simulink model "Md31StEnCtrl"  (R2018b)
settings: Solver=FixedStepDiscrete  StartTime=0.0  StopTime=10.0  FixedStep=0.01  RelTol=1e-3  EnableMultiTasking=on
undefined symbols (not defined in the file or in its folder): data, KeSMSuFirstRwStFwdBkwdPosDelta_Val, KeSMSw4SSecRwRtStLgrstOtwdInwdClosePos1_Val, KeSMSw4SSecRwRtStLgrstUpwdDnwdClosePos1_Val, KeSMSw4SSecRwRtStLgrstUpwdDnwdClosePos2_Val, PassStBkReclnEn_Clear, PassStBkReclnEn_Set, PassStCshnFldEn_Clear, PassStCshnFldEn_Set, PassStFwdBkwdEn_Clear, PassStFwdBkwdEn_Set, SecRwRtStLgrstInwdOtwdEn_Clear, SecRwRtStLgrstInwdOtwdEn_Set, SecRwRtStLgrstUpwdDnwdEn_Clear, SecRwRtStLgrstUpwdDnwdEn_Set
libraries: simulink x2
settings Model: Creator=sn55gm  LastModifiedBy=sn55gm
settings Model: ModifiedHistory=|
  | 2025.7.15 二排腿托enset修复
  | 2025.09.03 前后或折叠都fail结束执行
settings DataIOCC: SaveFormat=StructureWithTime
settings OptimizationCC: DefaultParameterBehavior=Inlined  UseDivisionForNetSlopeComputation=on  UseFloatMulNetSlope=on  InlineInvariantSignals=on  PassReuseOutputArgsAs=Individual arguments  ZeroExternalMemoryAtStartup=off  ZeroInternalMemoryAtStartup=off  NoFixptDivByZeroProtection=on  EfficientFloat2IntCast=on  LifeSpan=1  OptimizeBlockOrder=speed  DifferentSizesBufferReuse=on
settings DebuggingCC: ParameterTunabilityLossMsg=error
settings HardwareCC: ProdLongLongMode=on
settings SFSimCC: MATLABDynamicMemAlloc=off
settings RTWCC: SystemTargetFile=autosar.tlc  GenCodeOnly=on  TemplateMakefile=ert_default_tmf  Description=AUTOSAR  GenerateReport=on  IncludeHyperlinkInReport=on  LaunchReport=on  GenerateTraceInfo=on  GenerateTraceReport=on  GenerateTraceReportSl=on  GenerateTraceReportSf=on  GenerateTraceReportEml=on  GenerateCodeMetricsReport=on
settings CodeAppCC: ForceParamTrailComments=on  IgnoreCustomStorageClasses=off  OperatorAnnotations=on  SimulinkDataObjDesc=on  SFDataObjDesc=on  CustomSymbolStrGlobalVar=rt$N$M  CustomSymbolStrType=$N$M  CustomSymbolStrFcn=$N$M$F  CustomSymbolStrMacro=$N$M  InsertBlockDesc=on
settings STFCustomTargetCC: TargetLangStandard=C99 (ISO)  MultiwordLength=256  ParMdlRefBuildCompliant=on  CompOptLevelCompliant=on  IncludeMdlTerminateFcn=off  CombineOutputUpdateFcns=on  CombineSignalStateStructs=on  SuppressErrorStatus=on  ERTCustomFileBanners=on  SupportAbsoluteTime=off  SupportNonFinite=off  SupportComplex=off  SupportContinuousTime=off  SupportNonInlinedSFcns=off  RemoveResetFunc=on  MATLABClassNameForMDSCustomization=Simulink.SoftwareTarget.ERTCustomization  AutosarCompliant=on  UseToolchainInfoCompliant=on  LookupTableObjectStructAxisOrder=2,1,3,4,...  LUTObjectStructOrderEvenSpacing=Size,Table,Breakpoints  SystemTargetFile=autosar.tlc
settings ERTTargetCC: TargetLangStandard=C99 (ISO)  ConcurrentExecutionCompliant=off  IncludeMdlTerminateFcn=off  CombineSignalStateStructs=on  SuppressErrorStatus=on  SupportAbsoluteTime=off  SupportNonFinite=off  SupportComplex=off  ModelStepFunctionPrototypeControlCompliant=off  CPPClassGenCompliant=off  AutosarCompliant=on  LookupTableObjectStructAxisOrder=2,1,3,4,...  LUTObjectStructOrderEvenSpacing=Size,Table,Breakpoints  InlinedParameterPlacement=NonHierarchical  ERTCustomFileTemplate=example_file_process.tlc  ERTFilePackagingFormat=CompactWithDataFile

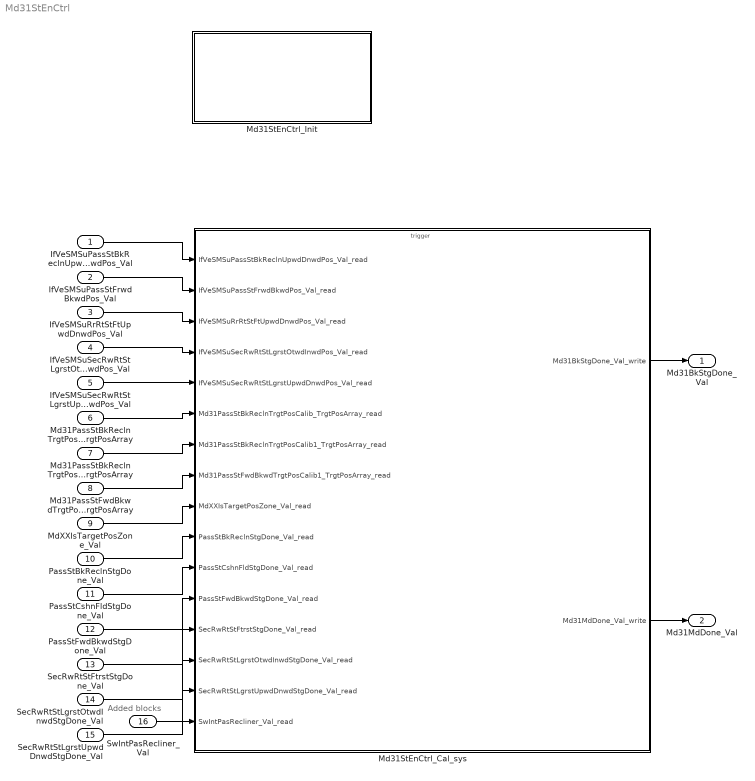
== system Md31StEnCtrl ==
  note: Added blocks
  IfVeSMSuPassStBkReclnUpwdDnwdPos_Val : Inport  OutDataTypeStr=uint16  PortDimensions=1
  IfVeSMSuPassStFrwdBkwdPos_Val : Inport  Port=2  OutDataTypeStr=uint16  PortDimensions=1
  IfVeSMSuRrRtStFtUpwdDnwdPos_Val : Inport  Port=3  OutDataTypeStr=uint16  PortDimensions=1
  IfVeSMSuSecRwRtStLgrstOtwdInwdPos_Val : Inport  Port=4  OutDataTypeStr=uint16  PortDimensions=1
  IfVeSMSuSecRwRtStLgrstUpwdDnwdPos_Val : Inport  Port=5  OutDataTypeStr=uint16  PortDimensions=1
  Md31PassStBkReclnTrgtPosCalib_TrgtPosArray : Inport  Description=|  Port=6  OutDataTypeStr=uint16  PortDimensions=3
      | 0:Pos
      | 1:Max
      | 2:Min
  Md31PassStBkReclnTrgtPosCalib1_TrgtPosArray : Inport  Description=|  Port=7  OutDataTypeStr=uint16  PortDimensions=3
      | 0:Pos
      | 1:Max
      | 2:Min
  Md31PassStFwdBkwdTrgtPosCalib1_TrgtPosArray : Inport  Description=|  Port=8  OutDataTypeStr=uint16  PortDimensions=3
      | 0:Pos
      | 1:Max
      | 2:Min
  MdXXIsTargetPosZone_Val : Inport  Port=9  OutDataTypeStr=uint32  PortDimensions=1
  PassStBkReclnStgDone_Val : Inport  Port=10  OutDataTypeStr=boolean  PortDimensions=1
  PassStCshnFldStgDone_Val : Inport  Port=11  OutDataTypeStr=boolean  PortDimensions=1
  PassStFwdBkwdStgDone_Val : Inport  Port=12  OutDataTypeStr=boolean  PortDimensions=1
  SecRwRtStFtrstStgDone_Val : Inport  Port=13  OutDataTypeStr=boolean  PortDimensions=1
  SecRwRtStLgrstOtwdInwdStgDone_Val : Inport  Port=14  OutDataTypeStr=boolean  PortDimensions=1
  SecRwRtStLgrstUpwdDnwdStgDone_Val : Inport  Port=15  OutDataTypeStr=boolean  PortDimensions=1
  SwIntPasRecliner_Val : Inport  Port=16  OutDataTypeStr=boolean  PortDimensions=1
  Md31StEnCtrl_Cal_sys : Subsystem
  Md31StEnCtrl_Init : Subsystem
  Md31BkStgDone_Val : Outport  OutDataTypeStr=boolean  PortDimensions=1
  Md31MdDone_Val : Outport  Port=2  OutDataTypeStr=uint8  PortDimensions=1
  wires:
  IfVeSMSuPassStBkReclnUpwdDnwdPos_Val/1 -> Md31StEnCtrl_Cal_sys/1(IfVeSMSuPassStBkReclnUpwdDnwdPos_Val_read)
  IfVeSMSuPassStFrwdBkwdPos_Val/1 -> Md31StEnCtrl_Cal_sys/2(IfVeSMSuPassStFrwdBkwdPos_Val_read)
  IfVeSMSuRrRtStFtUpwdDnwdPos_Val/1 -> Md31StEnCtrl_Cal_sys/3(IfVeSMSuRrRtStFtUpwdDnwdPos_Val_read)
  IfVeSMSuSecRwRtStLgrstOtwdInwdPos_Val/1 -> Md31StEnCtrl_Cal_sys/4(IfVeSMSuSecRwRtStLgrstOtwdInwdPos_Val_read)
  IfVeSMSuSecRwRtStLgrstUpwdDnwdPos_Val/1 -> Md31StEnCtrl_Cal_sys/5(IfVeSMSuSecRwRtStLgrstUpwdDnwdPos_Val_read)
  Md31PassStBkReclnTrgtPosCalib_TrgtPosArray/1 -> Md31StEnCtrl_Cal_sys/6(Md31PassStBkReclnTrgtPosCalib_TrgtPosArray_read)
  Md31PassStBkReclnTrgtPosCalib1_TrgtPosArray/1 -> Md31StEnCtrl_Cal_sys/7(Md31PassStBkReclnTrgtPosCalib1_TrgtPosArray_read)
  Md31PassStFwdBkwdTrgtPosCalib1_TrgtPosArray/1 -> Md31StEnCtrl_Cal_sys/8(Md31PassStFwdBkwdTrgtPosCalib1_TrgtPosArray_read)
  MdXXIsTargetPosZone_Val/1 -> Md31StEnCtrl_Cal_sys/9(MdXXIsTargetPosZone_Val_read)
  PassStBkReclnStgDone_Val/1 -> Md31StEnCtrl_Cal_sys/10(PassStBkReclnStgDone_Val_read)
  PassStCshnFldStgDone_Val/1 -> Md31StEnCtrl_Cal_sys/11(PassStCshnFldStgDone_Val_read)
  PassStFwdBkwdStgDone_Val/1 -> Md31StEnCtrl_Cal_sys/12(PassStFwdBkwdStgDone_Val_read)
  SecRwRtStFtrstStgDone_Val/1 -> Md31StEnCtrl_Cal_sys/13(SecRwRtStFtrstStgDone_Val_read)
  SecRwRtStLgrstOtwdInwdStgDone_Val/1 -> Md31StEnCtrl_Cal_sys/14(SecRwRtStLgrstOtwdInwdStgDone_Val_read)
  SecRwRtStLgrstUpwdDnwdStgDone_Val/1 -> Md31StEnCtrl_Cal_sys/15(SecRwRtStLgrstUpwdDnwdStgDone_Val_read)
  Md31StEnCtrl_Cal_sys/1(Md31BkStgDone_Val_write) -> Md31BkStgDone_Val/1
  Md31StEnCtrl_Cal_sys/2(Md31MdDone_Val_write) -> Md31MdDone_Val/1
  SwIntPasRecliner_Val/1 -> Md31StEnCtrl_Cal_sys/16(SwIntPasRecliner_Val_read)

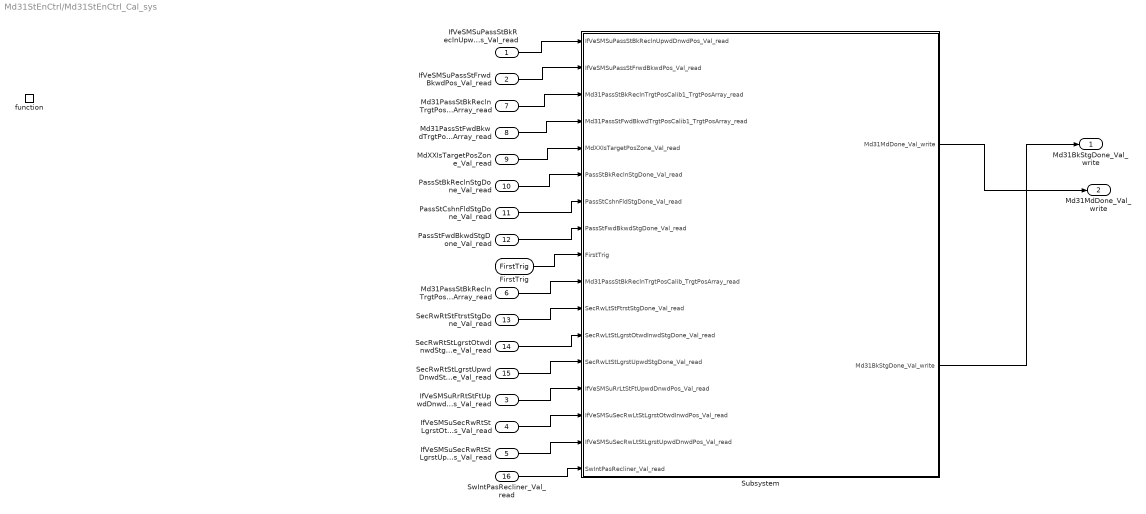
== system Md31StEnCtrl/Md31StEnCtrl_Cal_sys ==
  IfVeSMSuPassStBkReclnUpwdDnwdPos_Val_read : Inport
  IfVeSMSuPassStFrwdBkwdPos_Val_read : Inport  Port=2
  IfVeSMSuRrRtStFtUpwdDnwdPos_Val_read : Inport  Port=3
  IfVeSMSuSecRwRtStLgrstOtwdInwdPos_Val_read : Inport  Port=4
  IfVeSMSuSecRwRtStLgrstUpwdDnwdPos_Val_read : Inport  Port=5
  Md31PassStBkReclnTrgtPosCalib_TrgtPosArray_read : Inport  Port=6
  Md31PassStBkReclnTrgtPosCalib1_TrgtPosArray_read : Inport  Port=7
  Md31PassStFwdBkwdTrgtPosCalib1_TrgtPosArray_read : Inport  Port=8
  MdXXIsTargetPosZone_Val_read : Inport  Port=9
  PassStBkReclnStgDone_Val_read : Inport  Port=10
  PassStCshnFldStgDone_Val_read : Inport  Port=11
  PassStFwdBkwdStgDone_Val_read : Inport  Port=12
  SecRwRtStFtrstStgDone_Val_read : Inport  Port=13
  SecRwRtStLgrstOtwdInwdStgDone_Val_read : Inport  Port=14
  SecRwRtStLgrstUpwdDnwdStgDone_Val_read : Inport  Port=15
  SwIntPasRecliner_Val_read : Inport  Port=16
  function : TriggerPort  TriggerType=function-call  IsSimulinkFunction=on  FunctionName=Md31StEnCtrl_Cal  VariantControl=(inherit)
  Subsystem : Subsystem
  FirstTrig : ArgIn  OutDataTypeStr=boolean  ArgumentName=FirstTrig
  Md31BkStgDone_Val_write : Outport
      settings: EnsureOutportIsVirtual=on
  Md31MdDone_Val_write : Outport  Port=2
      settings: EnsureOutportIsVirtual=on
  wires:
  IfVeSMSuPassStBkReclnUpwdDnwdPos_Val_read/1 -> Subsystem/1(IfVeSMSuPassStBkReclnUpwdDnwdPos_Val_read)
  Md31PassStFwdBkwdTrgtPosCalib1_TrgtPosArray_read/1 -> Subsystem/4(Md31PassStFwdBkwdTrgtPosCalib1_TrgtPosArray_read)
  PassStBkReclnStgDone_Val_read/1 -> Subsystem/6(PassStBkReclnStgDone_Val_read)
  PassStFwdBkwdStgDone_Val_read/1 -> Subsystem/8(PassStFwdBkwdStgDone_Val_read)
  FirstTrig/1 -> Subsystem/9(FirstTrig)
  Subsystem/2(Md31BkStgDone_Val_write) -> Md31BkStgDone_Val_write/1
  Subsystem/1(Md31MdDone_Val_write) -> Md31MdDone_Val_write/1
  IfVeSMSuPassStFrwdBkwdPos_Val_read/1 -> Subsystem/2(IfVeSMSuPassStFrwdBkwdPos_Val_read)
  MdXXIsTargetPosZone_Val_read/1 -> Subsystem/5(MdXXIsTargetPosZone_Val_read)
  PassStCshnFldStgDone_Val_read/1 -> Subsystem/7(PassStCshnFldStgDone_Val_read)
  SecRwRtStFtrstStgDone_Val_read/1 -> Subsystem/11(SecRwLtStFtrstStgDone_Val_read)
  SecRwRtStLgrstOtwdInwdStgDone_Val_read/1 -> Subsystem/12(SecRwLtStLgrstOtwdInwdStgDone_Val_read)
  SecRwRtStLgrstUpwdDnwdStgDone_Val_read/1 -> Subsystem/13(SecRwLtStLgrstUpwdStgDone_Val_read)
  IfVeSMSuRrRtStFtUpwdDnwdPos_Val_read/1 -> Subsystem/14(IfVeSMSuRrLtStFtUpwdDnwdPos_Val_read)
  Md31PassStBkReclnTrgtPosCalib_TrgtPosArray_read/1 -> Subsystem/10(Md31PassStBkReclnTrgtPosCalib_TrgtPosArray_read)
  Md31PassStBkReclnTrgtPosCalib1_TrgtPosArray_read/1 -> Subsystem/3(Md31PassStBkReclnTrgtPosCalib1_TrgtPosArray_read)
  IfVeSMSuSecRwRtStLgrstOtwdInwdPos_Val_read/1 -> Subsystem/15(IfVeSMSuSecRwLtStLgrstOtwdInwdPos_Val_read)
  IfVeSMSuSecRwRtStLgrstUpwdDnwdPos_Val_read/1 -> Subsystem/16(IfVeSMSuSecRwLtStLgrstUpwdDnwdPos_Val_read)
  SwIntPasRecliner_Val_read/1 -> Subsystem/17(SwIntPasRecliner_Val_read)

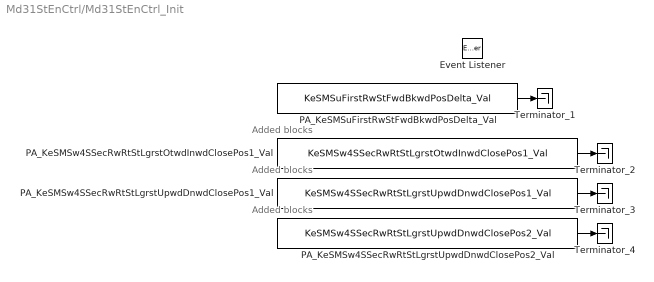
== system Md31StEnCtrl/Md31StEnCtrl_Init ==
  note: Added blocks
  note: Added blocks
  note: Added blocks
  Event Listener : EventListener  EventName=reset
  PA_KeSMSuFirstRwStFwdBkwdPosDelta_Val : Constant  Value=KeSMSuFirstRwStFwdBkwdPosDelta_Val
  PA_KeSMSw4SSecRwRtStLgrstOtwdInwdClosePos1_Val : Constant  Value=KeSMSw4SSecRwRtStLgrstOtwdInwdClosePos1_Val
  PA_KeSMSw4SSecRwRtStLgrstUpwdDnwdClosePos1_Val : Constant  Value=KeSMSw4SSecRwRtStLgrstUpwdDnwdClosePos1_Val
  PA_KeSMSw4SSecRwRtStLgrstUpwdDnwdClosePos2_Val : Constant  Value=KeSMSw4SSecRwRtStLgrstUpwdDnwdClosePos2_Val
  Terminator_{1..4} (4 alike) : Terminator
  wires:
  PA_KeSMSuFirstRwStFwdBkwdPosDelta_Val/1 -> Terminator_1/1
  PA_KeSMSw4SSecRwRtStLgrstOtwdInwdClosePos1_Val/1 -> Terminator_2/1
  PA_KeSMSw4SSecRwRtStLgrstUpwdDnwdClosePos1_Val/1 -> Terminator_3/1
  PA_KeSMSw4SSecRwRtStLgrstUpwdDnwdClosePos2_Val/1 -> Terminator_4/1

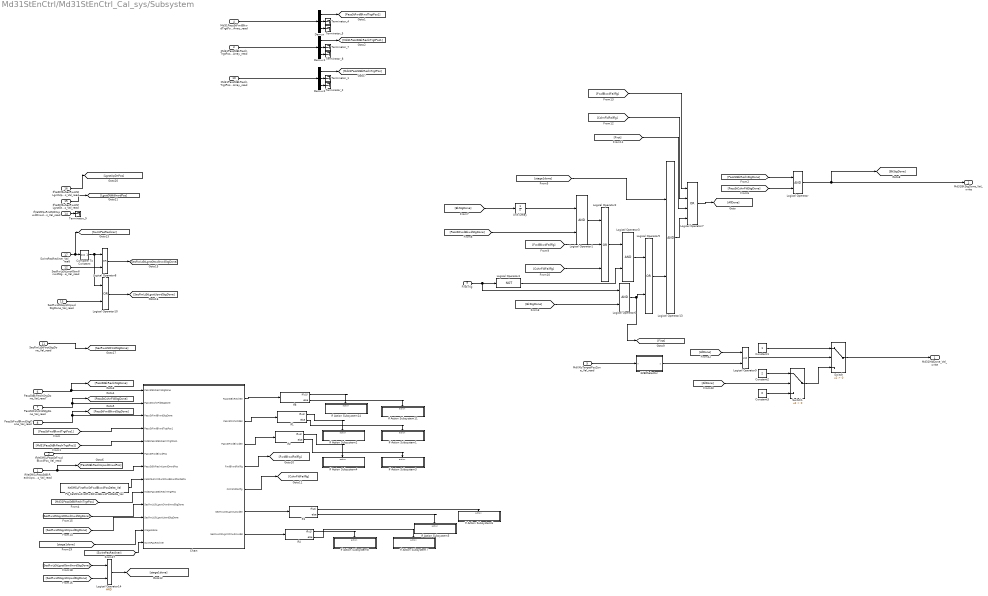
== system Md31StEnCtrl/Md31StEnCtrl_Cal_sys/Subsystem ==
  IfVeSMSuPassStBkReclnUpwdDnwdPos_Val_read : Inport
  IfVeSMSuPassStFrwdBkwdPos_Val_read : Inport  Port=2
  Md31PassStBkReclnTrgtPosCalib1_TrgtPosArray_read : Inport  Port=3
  Md31PassStFwdBkwdTrgtPosCalib1_TrgtPosArray_read : Inport  Port=4
  MdXXIsTargetPosZone_Val_read : Inport  Port=5
  PassStBkReclnStgDone_Val_read : Inport  Port=6
  PassStCshnFldStgDone_Val_read : Inport  Port=7
  PassStFwdBkwdStgDone_Val_read : Inport  Port=8
  FirstTrig : Inport  Port=9
  Md31PassStBkReclnTrgtPosCalib_TrgtPosArray_read : Inport  Port=10
  SecRwLtStFtrstStgDone_Val_read : Inport  Port=11
  SecRwLtStLgrstOtwdInwdStgDone_Val_read : Inport  Port=12
  SecRwLtStLgrstUpwdStgDone_Val_read : Inport  Port=13
  IfVeSMSuRrLtStFtUpwdDnwdPos_Val_read : Inport  Port=14
  IfVeSMSuSecRwLtStLgrstOtwdInwdPos_Val_read : Inport  Port=15
  IfVeSMSuSecRwLtStLgrstUpwdDnwdPos_Val_read : Inport  Port=16
  SwIntPasRecliner_Val_read : Inport  Port=17
  32BitSelector : Subsystem  mask(32 Bit Selector){BitNum=30}
      mask prompts: BitNum "Select Bit Number"
      mask help: Allows selection of a particular bit (0-31) out of a packed word up to 32 bits long. Output will be true if the bit number selected via the mask parameter is equal to one.
      mask TypeOptions BitNum: 0 | 1 | 2 | 3 | 4 | 5 | 6 | 7 | 8 | 9 | 10 | 11 | 12 | 13 | 14 | 15 | 16 | 17 | 18 | 19 | 20 | 21 | 22 | 23 | 24 | 25 | 26 | 27 | 28 | 29 | 30 | 31
      mask Display:
      | text(0.5, 0.8,'BIT','horizontalAlignment','center')
      | text(0.5, 0.5,'SELECTOR','horizontalAlignment','center')
      | text(0.5, 0.2,['-- Bit ',char(get_param(gcb,'BitNum')),' --'],'horizontalAlignment','center')
  Chart : Stateflow chart  TreatAsAtomicUnit=on
  Compare To Constant : simulink/Logic and Bit Operations/Compare To Constant  relop===  const=1  OutDataTypeStr=boolean
  Constant1 : Constant  OutDataTypeStr=uint8
  Constant2 : Constant  Value=2  OutDataTypeStr=uint8
  Constant3 : Constant  Value=0  OutDataTypeStr=uint8
  Demux : Demux  Outputs=3
  Demux1 : Demux  Outputs=3
  Demux2 : Demux  Outputs=3
  If Action Subsystem1 : Subsystem  TreatAsAtomicUnit=on
  If Action Subsystem11 : Subsystem  TreatAsAtomicUnit=on
  If Action Subsystem14 : Subsystem  TreatAsAtomicUnit=on
  If Action Subsystem2 : Subsystem  TreatAsAtomicUnit=on
  If Action Subsystem3 : Subsystem  TreatAsAtomicUnit=on
  If Action Subsystem4 : Subsystem  TreatAsAtomicUnit=on
  If Action Subsystem5 : Subsystem  TreatAsAtomicUnit=on
  If Action Subsystem6 : Subsystem  TreatAsAtomicUnit=on
  If Action Subsystem7 : Subsystem  TreatAsAtomicUnit=on
  If Action Subsystem8 : Subsystem  TreatAsAtomicUnit=on
  If{1..4,8} (5 alike) : If  IfExpression=u1
  Logical Operator{,1,3,6,9,13..14} (7 alike) : Logic  AllPortsSameDT=off  OutDataTypeStr=boolean
  Logical Operator10 : Logic  Operator=OR  AllPortsSameDT=off  OutDataTypeStr=boolean
  Logical Operator2 : Logic  Operator=OR  Inputs=3  AllPortsSameDT=off  OutDataTypeStr=boolean
  Logical Operator4 : Logic  Operator=NOT  AllPortsSameDT=off  OutDataTypeStr=boolean
  Logical Operator5 : Logic  Operator=OR  AllPortsSameDT=off  OutDataTypeStr=boolean
  Logical Operator7 : Logic  Operator=OR  Inputs=4  AllPortsSameDT=off  OutDataTypeStr=boolean
  Logical Operator8 : Logic  Operator=OR  AllPortsSameDT=off  OutDataTypeStr=boolean
  PA_KeSMSuFirstRwStFwdBkwdPosDelta_Val : Constant  Value=KeSMSuFirstRwStFwdBkwdPosDelta_Val
  Switch : Switch  Criteria=u2 > Threshold
  Switch1 : Switch  Criteria=u2 > Threshold
  Terminator_{1..2,4..5,7..9} (7 alike) : Terminator
  Unit Delay : UnitDelay  SampleTime=-1
  Md31MdDone_Val_write : Outport
      settings: EnsureOutportIsVirtual=on
  Md31BkStgDone_Val_write : Outport  Port=2
      settings: EnsureOutportIsVirtual=on
  wires:
  PA_KeSMSuFirstRwStFwdBkwdPosDelta_Val/1 -> Chart/8(KeSMSuFirstRwStFwdBkwdPosDelta)
  Constant2/1 -> Switch1/1
  Constant3/1 -> Switch1/3
  MdXXIsTargetPosZone_Val_read/1 -> 32BitSelector/1(x)
  Constant1/1 -> Switch/1
  [AllDone] -> Switch1/2
  Switch/1 -> Md31MdDone_Val_write/1
  [AllDone] -> Logical Operator9/1
  Logical Operator9/1 -> Switch/2
  Switch1/1 -> Switch/3
  If1/1 -> If Action Subsystem2/Action
  If2/1 -> If Action Subsystem4/Action
  If1/2 -> If Action Subsystem1/Action
  Chart/5(CshnFldFailflg) -> [CshnFldFailflg]
  If8/2 -> If Action Subsystem11/Action
  Chart/1(PassStBkReclnEn) -> If8/1
  Chart/4(FwdBkwdFailflg) -> [FwdBkwdFailflg]
  Chart/2(PassStCshnFldEn) -> If1/1
  If8/1 -> If Action Subsystem14/Action
  Chart/3(PassStFwdBkwdEn) -> If2/1
  If2/2 -> If Action Subsystem3/Action
  Demux1/3 -> Terminator_8/1
  Demux/2 -> Terminator_4/1
  Md31PassStBkReclnTrgtPosCalib1_TrgtPosArray_read/1 -> Demux1/1
  Md31PassStFwdBkwdTrgtPosCalib1_TrgtPosArray_read/1 -> Demux/1
  Demux1/2 -> Terminator_7/1
  Demux/3 -> Terminator_5/1
  Demux/1 -> [PassStFwdBkwdTrgtPos1]
  Demux1/1 -> [Md31PassStBkReclnTrgtPos1]
  PassStBkReclnStgDone_Val_read/1 -> [PassStBkReclnStgDone], Chart/1(PassStBkReclnStgDone)
  PassStCshnFldStgDone_Val_read/1 -> [PassStCshnFldStgDone], Chart/2(PassStCshnFldStgDone)
  PassStFwdBkwdStgDone_Val_read/1 -> [PassStFwdBkwdStgDone], Chart/3(PassStFwdBkwdStgDone)
  [PassStFwdBkwdTrgtPos1] -> Chart/4(PassStFwdBkwdTrgtPos1)
  [Md31PassStBkReclnTrgtPos1] -> Chart/5(Md31PassStBkReclnTrgtPos1)
  IfVeSMSuPassStFrwdBkwdPos_Val_read/1 -> Chart/6(PassStFwdBkwdPos)
  IfVeSMSuPassStBkReclnUpwdDnwdPos_Val_read/1 -> [PassStBkReclnUpwdDnwdPos], Chart/7(PassStBkReclnUpwdDnwdPos)
  Logical Operator/1 -> Md31BkStgDone_Val_write/1, [BkStgDone]
  [PassStCshnFldStgDone] -> Logical Operator/2
  Unit Delay/1 -> Logical Operator1/1
  Logical Operator1/1 -> Logical Operator2/1
  [PassStFwdBkwdStgDone] -> Logical Operator1/2
  [CshnFldFailflg] -> Logical Operator2/3
  [BkStgDone] -> Unit Delay/1
  [FwdBkwdFailflg] -> Logical Operator2/2
  32BitSelector/1(y) -> Logical Operator9/2
  [PassStBkReclnStgDone] -> Logical Operator/1
  Demux2/1 -> [Md31PassStBkReclnTrgtPos]
  Demux2/2 -> Terminator_1/1
  Md31PassStBkReclnTrgtPosCalib_TrgtPosArray_read/1 -> Demux2/1
  Demux2/3 -> Terminator_2/1
  [Md31PassStBkReclnTrgtPos] -> Chart/9(Md31PassStBkReclnTrgtPos)
  Logical Operator2/1 -> Logical Operator3/1
  FirstTrig/1 -> Logical Operator6/1, Logical Operator4/1
  Logical Operator4/1 -> Logical Operator3/2
  Logical Operator3/1 -> Logical Operator5/1
  Logical Operator6/1 -> [First], Logical Operator5/2
  [BkStgDone] -> Logical Operator6/2
  IfVeSMSuSecRwLtStLgrstUpwdDnwdPos_Val_read/1 -> [LgrstUpDnPos]
  IfVeSMSuSecRwLtStLgrstOtwdInwdPos_Val_read/1 -> [LgrstOtWdInwdPos]
  SecRwLtStFtrstStgDone_Val_read/1 -> [SecRwLtStFtrstStgDone]
  [stage1done] -> Logical Operator13/1
  Logical Operator5/1 -> Logical Operator13/2
  [SecRwLtStLgrstOtwdInwdStgDone] -> Chart/10(SecRwLtStLgrstOtwdInwdStgDone)
  [SecRwLtStLgrstUpwdStgDone] -> Chart/11(SecRwLtStLgrstUpwdStgDone)
  If3/1 -> If Action Subsystem6/Action
  If3/2 -> If Action Subsystem5/Action
  If4/1 -> If Action Subsystem8/Action
  If4/2 -> If Action Subsystem7/Action
  Chart/7(SecRwLtStLgrstOtwdInwdEn) -> If4/1
  Chart/6(SecRwLtStLgrstUpwdEn) -> If3/1
  [SecRwLtStLgrstOtwdInwdStgDone] -> Logical Operator14/1
  [SecRwLtStLgrstUpwdStgDone] -> Logical Operator14/2
  Logical Operator14/1 -> [stage1done]
  [stage1done] -> Chart/12(stage1done)
  Logical Operator13/1 -> Logical Operator7/4
  [First] -> Logical Operator7/3
  Logical Operator7/1 -> [AllDone]
  [CshnFldFailflg] -> Logical Operator7/2
  [FwdBkwdFailflg] -> Logical Operator7/1
  IfVeSMSuRrLtStFtUpwdDnwdPos_Val_read/1 -> Terminator_9/1
  SwIntPasRecliner_Val_read/1 -> [SwIntPasRecliner], Compare To Constant/1
  Compare To Constant/1 -> Logical Operator10/1, Logical Operator8/1
  Logical Operator8/1 -> [SecRwLtStLgrstOtwdInwdStgDone]
  SecRwLtStLgrstOtwdInwdStgDone_Val_read/1 -> Logical Operator8/2
  SecRwLtStLgrstUpwdStgDone_Val_read/1 -> Logical Operator10/2
  Logical Operator10/1 -> [SecRwLtStLgrstUpwdStgDone]
  [SwIntPasRecliner] -> Chart/13(SwIntPasRecliner)

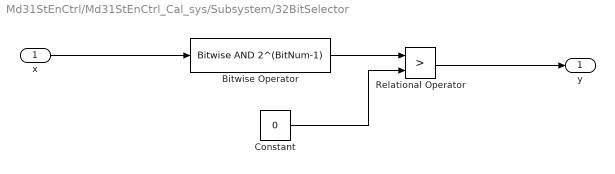
== system Md31StEnCtrl/Md31StEnCtrl_Cal_sys/Subsystem/32BitSelector ==
  x : Inport
  Bitwise Operator : simulink/Logic and Bit Operations/Bitwise Operator  logicop=AND  UseBitMask=on  BitMask=2^(BitNum-1)  BitMaskRealWorld=Stored Integer
  Constant : Constant  Value=0  OutDataTypeStr=uint32
  Relational Operator : RelationalOperator  Operator=>  OutDataTypeStr=boolean  RndMeth=Simplest
  y : Outport
  wires:
  Relational Operator/1 -> y/1
  Constant/1 -> Relational Operator/2
  x/1 -> Bitwise Operator/1
  Bitwise Operator/1 -> Relational Operator/1

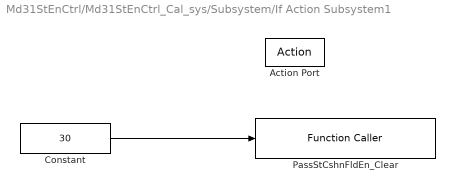
== system Md31StEnCtrl/Md31StEnCtrl_Cal_sys/Subsystem/If Action Subsystem1 ==
  Action Port : ActionPort  ActionType=else
  Constant : Constant  Value=30  OutDataTypeStr=uint8
  PassStCshnFldEn_Clear : FunctionCaller  FunctionPrototype=PassStCshnFldEn_Clear(data)  InputArgumentSpecifications=uint8(1)
  wires:
  Constant/1 -> PassStCshnFldEn_Clear/1

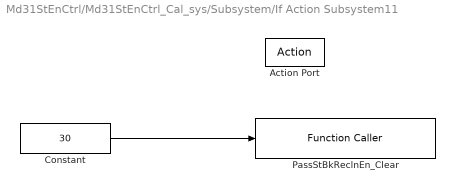
== system Md31StEnCtrl/Md31StEnCtrl_Cal_sys/Subsystem/If Action Subsystem11 ==
  Action Port : ActionPort  ActionType=else
  Constant : Constant  Value=30  OutDataTypeStr=uint8
  PassStBkReclnEn_Clear : FunctionCaller  FunctionPrototype=PassStBkReclnEn_Clear(data)  InputArgumentSpecifications=uint8(1)
  wires:
  Constant/1 -> PassStBkReclnEn_Clear/1

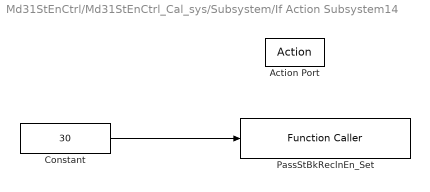
== system Md31StEnCtrl/Md31StEnCtrl_Cal_sys/Subsystem/If Action Subsystem14 ==
  Action Port : ActionPort  ActionType=then
  Constant : Constant  Value=30  OutDataTypeStr=uint8
  PassStBkReclnEn_Set : FunctionCaller  FunctionPrototype=PassStBkReclnEn_Set(data)  InputArgumentSpecifications=uint8(1)
  wires:
  Constant/1 -> PassStBkReclnEn_Set/1

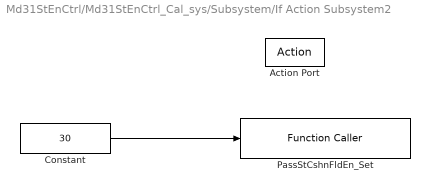
== system Md31StEnCtrl/Md31StEnCtrl_Cal_sys/Subsystem/If Action Subsystem2 ==
  Action Port : ActionPort  ActionType=then
  Constant : Constant  Value=30  OutDataTypeStr=uint8
  PassStCshnFldEn_Set : FunctionCaller  FunctionPrototype=PassStCshnFldEn_Set(data)  InputArgumentSpecifications=uint8(1)
  wires:
  Constant/1 -> PassStCshnFldEn_Set/1

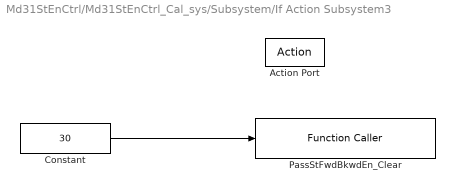
== system Md31StEnCtrl/Md31StEnCtrl_Cal_sys/Subsystem/If Action Subsystem3 ==
  Action Port : ActionPort  ActionType=else
  Constant : Constant  Value=30  OutDataTypeStr=uint8
  PassStFwdBkwdEn_Clear : FunctionCaller  FunctionPrototype=PassStFwdBkwdEn_Clear(data)  InputArgumentSpecifications=uint8(1)
  wires:
  Constant/1 -> PassStFwdBkwdEn_Clear/1

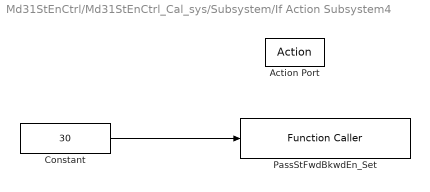
== system Md31StEnCtrl/Md31StEnCtrl_Cal_sys/Subsystem/If Action Subsystem4 ==
  Action Port : ActionPort  ActionType=then
  Constant : Constant  Value=30  OutDataTypeStr=uint8
  PassStFwdBkwdEn_Set : FunctionCaller  FunctionPrototype=PassStFwdBkwdEn_Set(data)  InputArgumentSpecifications=uint8(1)
  wires:
  Constant/1 -> PassStFwdBkwdEn_Set/1

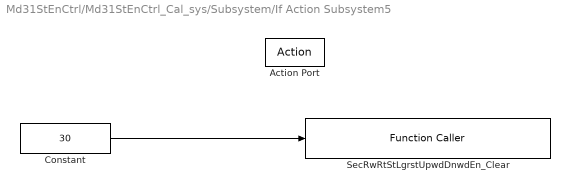
== system Md31StEnCtrl/Md31StEnCtrl_Cal_sys/Subsystem/If Action Subsystem5 ==
  Action Port : ActionPort  ActionType=else
  Constant : Constant  Value=30  OutDataTypeStr=uint8
  SecRwRtStLgrstUpwdDnwdEn_Clear : FunctionCaller  FunctionPrototype=SecRwRtStLgrstUpwdDnwdEn_Clear(data)  InputArgumentSpecifications=uint8(1)
  wires:
  Constant/1 -> SecRwRtStLgrstUpwdDnwdEn_Clear/1

== system Md31StEnCtrl/Md31StEnCtrl_Cal_sys/Subsystem/If Action Subsystem6 ==
  Action Port : ActionPort  ActionType=then
  Constant : Constant  Value=30  OutDataTypeStr=uint8
  SecRwRtStLgrstUpwdDnwdEn_Set : FunctionCaller  FunctionPrototype=SecRwRtStLgrstUpwdDnwdEn_Set(data)  InputArgumentSpecifications=uint8(1)
  wires:
  Constant/1 -> SecRwRtStLgrstUpwdDnwdEn_Set/1

== system Md31StEnCtrl/Md31StEnCtrl_Cal_sys/Subsystem/If Action Subsystem7 ==
  Action Port : ActionPort  ActionType=else
  Constant : Constant  Value=30  OutDataTypeStr=uint8
  SecRwRtStLgrstInwdOtwdEn_Clear : FunctionCaller  FunctionPrototype=SecRwRtStLgrstInwdOtwdEn_Clear(data)  InputArgumentSpecifications=uint8(1)
  wires:
  Constant/1 -> SecRwRtStLgrstInwdOtwdEn_Clear/1

== system Md31StEnCtrl/Md31StEnCtrl_Cal_sys/Subsystem/If Action Subsystem8 ==
  Action Port : ActionPort  ActionType=then
  Constant : Constant  Value=30  OutDataTypeStr=uint8
  SecRwRtStLgrstInwdOtwdEn_Set : FunctionCaller  FunctionPrototype=SecRwRtStLgrstInwdOtwdEn_Set(data)  InputArgumentSpecifications=uint8(1)
  wires:
  Constant/1 -> SecRwRtStLgrstInwdOtwdEn_Set/1

== stateflow chart Md31StEnCtrl/Md31StEnCtrl_Cal_sys/Subsystem/Chart ==
  (default) -> (junction 70) : {
      | PassStFwdBkwdEn = 0;
      | PassStBkReclnEn = 0;
      | PassStCshnFldEn = 0;
      | FwdBkwdFailflg = 0;
      | CshnFldFailflg = 0;
      | SecRwLtStLgrstUpwdEn=0;
      | SecRwLtStLgrstOtwdInwdEn=0;
      | }
  (junction 70) -> (junction 91) [order 1] : [SecRwLtStLgrstOtwdInwdStgDone]
  (junction 70) -> (junction 83) [order 2] : {SecRwLtStLgrstOtwdInwdEn=1;}
  (junction 91) -> (junction 92)
  (junction 92) -> (junction 83)
  (junction 83) -> (junction 84)
  (junction 84) -> (junction 95) [order 1] : [SecRwLtStLgrstUpwdStgDone]
  (junction 84) -> (junction 89) [order 2] : {SecRwLtStLgrstUpwdEn=1;}
  (junction 95) -> (junction 97)
  (junction 97) -> (junction 89)
  (junction 89) -> (junction 10)
  (junction 10) -> (junction 12) [order 1] : [PassStFwdBkwdStgDone]
  (junction 12) -> (junction 25) [order 1] : [(PassStFwdBkwdPos<(PassStFwdBkwdTrgtPos1-KeSMSuFirstRwStFwdBkwdPosDelta))&&(PassStBkReclnUpwdDnwdPos<=(Md31PassStBkReclnTrgtPos-120))]
  (junction 10) -> (junction 107) [order 2]
  (junction 12) -> (junction 16) [order 2]
  (junction 25) -> (junction 27) : {FwdBkwdFailflg =1;}
  (junction 107) -> (junction 109) [order 1] : [!stage1done&&SwIntPasRecliner==0]
  (junction 107) -> (junction 18) [order 2] : {PassStFwdBkwdEn = 1;}
  (junction 109) -> (junction 111)
  (junction 111) -> (junction 18)
  (junction 16) -> (junction 111)
  (junction 27) -> (junction 16)
  (junction 18) -> (junction 24)
  (junction 24) -> (junction 31) [order 1] : [stage1done&&...
      | PassStFwdBkwdStgDone &&...
      | (PassStFwdBkwdPos>=(PassStFwdBkwdTrgtPos1-KeSMSuFirstRwStFwdBkwdPosDelta)||...
      | PassStBkReclnUpwdDnwdPos>(Md31PassStBkReclnTrgtPos-120))]
  (junction 31) -> (junction 33) [order 1] : [PassStBkReclnStgDone ]
  (junction 33) -> (junction 56) [order 1] : [PassStBkReclnUpwdDnwdPos <Md31PassStBkReclnTrgtPos1]
  (junction 24) -> (junction 52) [order 2]
  (junction 31) -> (junction 35) [order 2] : {
      | PassStBkReclnEn = 1;
      | }
  (junction 33) -> (junction 40) [order 2]
  (junction 56) -> (junction 58) : {
      | CshnFldFailflg = 1;
      | }
  (junction 40) -> (junction 35)
  (junction 35) -> (junction 43)
  (junction 43) -> (junction 45) [order 1] : [(PassStBkReclnUpwdDnwdPos >=Md31PassStBkReclnTrgtPos1)&&!PassStCshnFldStgDone]
  (junction 43) -> (junction 49) [order 2]
  (junction 45) -> (junction 47) : {PassStCshnFldEn = 1;}
  (junction 49) -> (junction 52)
  (junction 47) -> (junction 49)
  (junction 58) -> (junction 47)
  (junction 52) -> (junction 103)
  data: PassStBkReclnStgDone input; PassStCshnFldStgDone input; PassStFwdBkwdStgDone input; PassStFwdBkwdTrgtPos1 input; Md31PassStBkReclnTrgtPos1 input; PassStFwdBkwdPos input; PassStBkReclnUpwdDnwdPos input; PassStBkReclnEn output boolean; PassStCshnFldEn output boolean; PassStFwdBkwdEn output boolean; FwdBkwdFailflg output boolean; CshnFldFailflg output boolean; KeSMSuFirstRwStFwdBkwdPosDelta input; Md31PassStBkReclnTrgtPos input; SecRwLtStLgrstOtwdInwdStgDone input; SecRwLtStLgrstUpwdStgDone input; SecRwLtStLgrstUpwdEn output boolean; SecRwLtStLgrstOtwdInwdEn output boolean; stage1done input; SwIntPasRecliner input
